simulink library "dspadpt3"  (Simulink 6.0)
settings: Solver=ode45  SolverMode=SingleTasking  StartTime=0.0  StopTime=10.0  RelTol=1e-3
undefined symbols (not defined in the file or in its folder): D, ic
libraries: dspsigattribs x27, dspmtrx3 x5, simulink x4, dspbuff3 x3, dspobslib x2, dspsigops x2, adptfiltsubsys x1, dspindex x1
settings Model: RequirementInfo=9  Creator=don  LastModifiedBy=mlongfri  ExtModeAutoUpdateStatusClock=off
settings Model: ForwardingTableString=|
  | ||__slOldName__||dspadpt3/RLS
  | Adaptive Filter||__slNewName__||dspobslib/RLS
  | Adaptive Filter||__slOldName__||dspadpt3/LMS
  | Adaptive Filter||__slNewName__||dspobslib/LMS
  | Adaptive Filter
settings DataIOCC: SignalLoggingName=logsOut
settings OptimizationCC: BooleanDataType=off
settings DebuggingCC: CheckExecutionContextPreStartOutputMsg=on  CheckExecutionContextRuntimeOutputMsg=on  SolverPrmCheckMsg=none
settings HardwareCC: TargetUnknown=on
settings ModelReferenceCC: UpdateModelReferenceTargets=IfOutOfDate
settings SFSimCC: SFSimApplyToAllLibs=on  SFSimBuildMode=Incremental

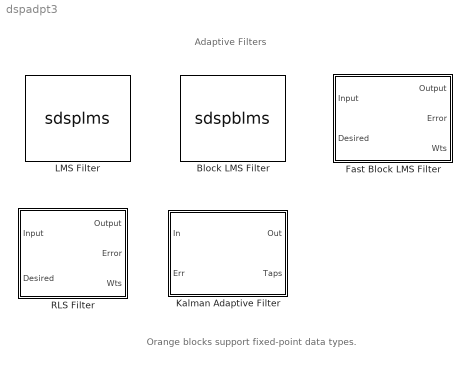
== system dspadpt3 ==
  note: Adaptive Filters
  note: Orange blocks support fixed-point data types.
  Block LMS Filter : S-Function  FunctionName=sdspblms  Parameters=L,N,stepflag,mu,leakage,addnparflag,ic,Adapt,resetflag,weights  mask(Block LMS Filter){algo=Block LMS, ShowPortLabels=off, L=32, N=32, stepflag=Dialog, mu=0.1, leakage=1.0, addnparflag=off, ic=0, Adapt=off, resetflag=None, weights=on}
      mask prompts: algo "dummy1"; ShowPortLabels "dummy2"; L "Filter length:"; N "Block size:"; stepflag "Specify step size via:"; mu "Step size (mu):"; leakage "Leakage factor (0 to 1):"; addnparflag "------------------------- Show additional parameters -------------------------"; ic "Initial value of filter weights:"; Adapt "Enable/disable adaptation via input port"; resetflag "Reset input:"; weights "Output filter weights"
      mask help:
      | Computes filter weights based on the Block LMS algorithm for filtering of the input signal. The filter weights are updated once for every block of data that is processed.
      |
      | Select the Enable/disable adaptation via input port check box to create an Adapt port on the block. When the input to this port is nonzero, the block continuously updates the filter weights. When the input to this port is zero, the filter weights remain constant.
      |
      | If the Reset port is enabled and a reset event occurs, the block resets the filter weights to their initial values.
      mask init:
      | resetflag = resetflag-1;
      | [si,so]=dspblkblklms('icon');
      | blkname = strvcat('  Block  ', '   LMS');
      mask Help: web(dspbhelp);
      mask StyleString: popup(Block LMS|Fast Block LMS),checkbox,edit,edit,popup(Dialog|Input port),edit,edit,checkbox,edit,checkbox,popup(None|Rising edge|Falling edge|Either edge|Non-zero sample),checkbox
      mask CallbackString: ||||dspblkblklms;|||dspblkblklms;||||
      mask Display:
      | disp(blkname)
      | port_label('input',si(1).port, si(1).txt);
      | port_label('input',si(2).port, si(2).txt);
      | port_label('input',si(3).port, si(3).txt);
      | port_label('input',si(4).port, si(4).txt);
      | port_label('input',si(5).port, si(5).txt);
      | 
      | port_label('output',so(1).port, so(1).txt);
      | port_label('output',so(2).port, so(2).txt);
      | port_label('output',so(3).port, so(3).txt);
  Fast Block LMS Filter : Subsystem  PropExecContextAcrossSSBoundary=on  mask(Fast Block LMS Filter){algo=Fast Block LMS, L=32, N=32, stepflag=Dialog, mu=0.1, leakage=1.0, addnparflag=off, ic=0, Adapt=off, resetflag=None, weights=on}
      mask prompts: algo "Algorithm:"; L "Filter length:"; N "Block size:"; stepflag "Specify step size via:"; mu "Step size (mu):"; leakage "Leakage factor (0 to 1):"; addnparflag "------------------------- Show additional parameters -------------------------"; ic "Inital value of filter weights:"; Adapt "Enable/disable adaptation via input port"; resetflag "Reset input:"; weights "Output filter weights"
      mask help:
      | Computes filter weights based on the Fast Block LMS algorithm for filtering of the input signal. The filter weights are updated once for every block of data that is processed. This block uses FFT for fast convolution.
      |
      | Select the Enable/disable adaptation via input port check box to create an Adapt port on the block. When the input to this port is nonzero, the block continuoulsy updates the filter weights. When the input to this port is zero, the filter weights remain constant.
      |
      | If the Reset port is enabled and a reset event occurs, the block resets the filter weights to their initial values.
      mask init:
      | if algo == 1
      | 	blkname = strvcat('  Block  ', '   LMS');
      | else
      | 	blkname = strvcat('Fast Block ', '    LMS');	
      | end
      | dspblkfblms('init');
      settings: ErrorFcn=dspblkadpterrfcn
      mask StyleString: popup(Block LMS|Fast Block LMS),edit,edit,popup(Dialog|Input port),edit,edit,checkbox,edit,checkbox,popup(None|Rising Edge|Falling Edge|Either Edge|Non-zero sample),checkbox
      mask CallbackString: |||dspblkfblms('addparams');|||dspblkfblms('addparams');||||
      mask Display: disp(blkname);
  Kalman Adaptive Filter : Subsystem  PropExecContextAcrossSSBoundary=on  mask(Kalman Adaptive Filter){Ntaps=64, Jmin=0.3, q=0.1, ic0=0, K0=0.5, Adapt=off, RstPort=None}
      mask prompts: Ntaps "FIR filter length:"; Jmin "Measurement noise variance:"; q "Process noise variance:"; ic0 "Initial value of filter taps:"; K0 "Initial error correlation matrix:"; Adapt "Adapt input"; RstPort "Reset input:"
      mask help:
      | One-step Kalman predictor algorithm for adaptive FIR filtering of input signal.
      |
      | If 'Adapt input' is checked and the Adapt signal is zero, the algorithm temporarily disables adaptation of the filter coefficients.  A non-zero signal enables filter adaptation.
      |
      | If the 'Reset input' is enabled and the Reset signal transitions appropriately, the filter coefficients are reset to the initial conditions.
      mask init:
      | if prod(size(ic0))==1, ic = ic0(ones(Ntaps,1)); else ic = ic0; end
      | if prod(size(K0))==1, K = K0.*eye(Ntaps);
      | elseif any(size(K0)==1), K = diag(K0);
      | else K=K0; end
      | dspblkadpt('init');
      mask Help: web(dspbhelp);
      mask StyleString: edit,edit,edit,edit,edit,checkbox,popup(None|Rising edge|Falling edge|Either edge|Non-zero sample)
      mask Display: disp('Kalman')
  LMS Filter : S-Function  DialogController=dspDDGCreate  DialogControllerArgs=DataTag0  FunctionName=sdsplms  Parameters=Algo,L,stepflag,mu,leakage,ic,Adapt,resetflag,weights,accum2Mode,accum2FracLength,prodOutput2Mode,prodOutput2FracLength,prodOutput3Mode,prodOutput3FracLength,prodOutput4Mode,prodOutput4FracLength,quotientMode,quotientFracLength,dtInfo.firstCoeffMode, dtInfo.firstCoeffWordLength, dtInfo.firstCoeffFracLength,dtInfo.firstCoeffMode, dtInfo.firstCoeffWordLength, dtInfo.secondCoeffFracLength,dtInfo.prodOutputMode,dtInfo.prodOutputWordLength,dtInfo.prodOutputFracLength,dtInfo.accumMode,dtInfo.accumWordLength,dtInfo.accumFracLength,dtInfo.memoryMode,dtInfo.memoryWordLength,dtInfo.memoryFracLength,dtInfo.roundingMode,dtInfo.overflowMode  mask(LMS Filter){ShowPortLabels=off, Algo=LMS, L=32, stepflag=Dialog, mu=0.1, leakage=1.0, ic=0, Adapt=off, resetflag=None, weights=on, firstCoeffMode=Same word length as first input, firstCoeffWordLength=16, firstCoeffFracLength=15, secondCoeffMode=User-defined, secondCoeffWordLength=2, secondCoeffFracLength=15, accumMode=Same as first input, accumWordLength=32, accumFracLength=20, accum2Mode=User-defined, accum2FracLength=20, prodOutputMode=Same as first input, prodOutputWordLength=32, prodOutputFracLength=20, prodOutput2Mode=User-defined, prodOutput2FracLength=20, prodOutput3Mode=User-defined, prodOutput3FracLength=20, prodOutput4Mode=User-defined, prodOutput4FracLength=20, quotientMode=User-defined, quotientFracLength=20, memoryMode=Same as first input, memoryWordLength=16, memoryFracLength=15, roundingMode=Floor, overflowMode=off, addnparflag=off}
      mask prompts: ShowPortLabels "dummy"; Algo "Algorithm:"; L "Filter length:"; stepflag "Specify step size via:"; mu "Step size (mu):"; leakage "Leakage factor (0 to 1):"; ic "Initial value of filter weights:"; Adapt "Enable/disable adaptation via input port"; resetflag "Reset input:"; weights "Output filter weights"; firstCoeffMode "Step size (mu) attributes:"; firstCoeffWordLength "Step size (mu) word length:"; firstCoeffFracLength "Step size (mu) fraction length:"; secondCoeffMode "Leakage factor attributes:"; secondCoeffWordLength "DUMMY lkg wordlength:"; secondCoeffFracLength "Leakage factor fraction length:"; accumMode "Accumulator (XTX) attributes:"; accumWordLength "Accumulator (XTX) word length:"; accumFracLength "Accumulator (XTX) fraction length:"; accum2Mode "Accumulator (WTX) attributes:"; accum2FracLength "Accumulator (WTX) fraction length:"; prodOutputMode "Product (XTX) output attributes:"; prodOutputWordLength "Product (XTX) output word length:"; prodOutputFracLength "Product (XTX) output fraction length:"; prodOutput2Mode "Product (WTX) output attributes:"; prodOutput2FracLength "Product (WTX) output fraction length:"; prodOutput3Mode "Product (mu*e) output attributes:"; prodOutput3FracLength "Product (mu*e) output fraction length:"; prodOutput4Mode "Product (Q*x) output attributes:"; prodOutput4FracLength "Product (Q*x) output fraction length:"; quotientMode "Quotient attributes:"; quotientFracLength "Quotient fraction length:"; memoryMode "State memory attributes:"; memoryWordLength "State memory word length:"; memoryFracLength "State memory fraction length:"; roundingMode "Round integer calculations toward:"; overflowMode "Saturate on integer overflow"; addnparflag "Dummy parameter"
      mask help:
      | Adapts the filter weights based on the chosen algorithm for filtering of the input signal.
      |
      | Select the Enable/disable adaptation via input port check box to create an Adapt port on the block. When the input to this port is nonzero, the block continuously updates the filter weights. When the input to this port is zero, the filter weights remain constant.
      |
      | If the Reset port is enabled and a reset event occurs, the block resets the filter weights to their initial values.
      mask init:
      | resetflag = resetflag-1;
      | ic=flipud(ic(:));
      | [si,so,disp_str,dtInfo]=dspblklms;
      | 
      | SAME_AS = 1;
      | USER_DEF = 2;
      | % prod outputs
      | if dtInfo.prodOutputMode == 0 % 'USER_DEFINED'
      | 	prodOutput2Mode = USER_DEF;
      | 	prodOutput3Mode = USER_DEF;
      | 	prodOutput4Mode = USER_DEF;
      | 	quotientMode = USER_DEF;
      | else
      | 	prodOutput2Mode = SAME_AS;
      | 	prodOutput3Mode = SAME_AS;
      | 	prodOutput4Mode = SAME_AS;
      | 	quotientMode = SAME_AS;
      | end
      | 	
      | % accums
      | if dtInfo.accumMode == 0 % 'USER_DEFINED'
      | 	accum2Mode = USER_DEF;
      | else
      | 	accum2Mode = SAME_AS;
      | end
      settings: CopyFcn=dspfixptcopycallback;
      mask Help: web(dspbhelp);
      mask StyleString: checkbox,popup(LMS|Normalized LMS|Sign-Error LMS|Sign-Data LMS|Sign-Sign LMS),edit,popup(Dialog|Input port),edit,edit,edit,checkbox,popup(None|Rising edge|Falling edge|Either edge|Non-zero sample),checkbox,popup(Same word length as first input|Specify word length|Binary point scaling|Slope and bias scaling|User-defined),edit,edit,popup(Same word length as first input|Specify word length|Binary point scaling|Slope and bias scaling|User-defined),edit,edit,popup(Same as first input|Binary point scaling|Slope and bias scaling|User-defined),edit,edit,popup(Same as first accumulator|Binary point scaling|Slope and bias scaling|User-defined),edit,popup(Same as first input|Binary point scaling|Slope and bias scaling|User-defined),edit,edit,popup(Same as first product|Binary point scaling|Slope and bias scaling|User-defined),edit,popup(Same as first product|Binary point scaling|Slope and bias scaling|User-defined),edit,popup(Same as first product|Binary point scaling|Slope and bias scaling|User-defined),edit,popup(Same as first product|Binary point scaling|Slope and bias scaling|User-defined),edit,popup(Same as first input|Binary point scaling|Slope and bias scaling|User-defined),edit,edit,popup(Floor|Nearest),checkbox,checkbox
      mask Display:
      | disp(disp_str)
      | port_label('input',si(1).port, si(1).txt);
      | port_label('input',si(2).port, si(2).txt);
      | port_label('input',si(3).port, si(3).txt);
      | port_label('input',si(4).port, si(4).txt);
      | port_label('input',si(5).port, si(5).txt);
      | 
      | port_label('output',so(1).port, so(1).txt);
      | port_label('output',so(2).port, so(2).txt);
      | port_label('output',so(3).port, so(3).txt);
  RLS Filter : Subsystem  PropExecContextAcrossSSBoundary=on  mask(RLS Adaptive filter){L=32, lambdaflag=Dialog, lambda=1.0, addnparflag=off, ic=0, delta=0.1, Adapt=off, resetflag=None, weights=on}
      mask prompts: L "Filter length:"; lambdaflag "Specify forgetting factor via:"; lambda "Forgetting factor (0 to 1):"; addnparflag "------------------------- Show additional parameters -------------------------"; ic "Initial value of filter weights:"; delta "Initial input variance estimate:"; Adapt "Enable/disable adaptation via input port"; resetflag "Reset input:"; weights "Output filter weights"
      mask help:
      | Computes filter weights based on the exponentially weighted recursive least-squares (RLS) algorithm for adaptive filtering of the input signal.
      |
      | Select the Enable/disable adaptation via input port check box to create an Adapt port on the block. When the input to this port is nonzero, the block continuoulsy updates the filter weights. When the input to this port is zero, the filter weights remain constant.
      |
      | If the Reset port is enabled and a reset event occurs, the block resets the filter weights to their initial values.
      mask init:
      | s ='RLS';
      | dspblkrls('init');
      settings: ErrorFcn=dspblkadpterrfcn
      mask StyleString: edit,popup(Dialog|Input port),edit,checkbox,edit,edit,checkbox,popup(None|Rising edge|Falling edge|Either edge|Non-zero sample),checkbox
      mask CallbackString: |dspblkrls('addparams');||dspblkrls('addparams');|||||
      mask Display: disp(s);

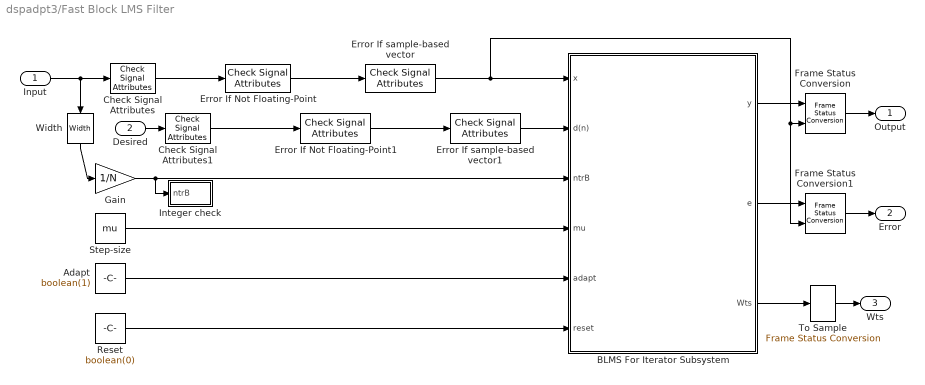
== system dspadpt3/Fast Block LMS Filter ==
  Input : Inport  LatchInput=off
  Desired : Inport  Port=2  LatchInput=off
  Adapt : Constant  Value=boolean(1)
  BLMS For Iterator Subsystem : Subsystem  TreatAsAtomicUnit=on  PropExecContextAcrossSSBoundary=on  mask{algo_for=Fast Block LMS, stepflag_for=off, weights_for=on}
      mask prompts: algo_for "Algorithm:"; stepflag_for "Input step size via port:"; weights_for "Send filter weights to output:"
      mask init:
      | dspblkfblmsfor;
      mask StyleString: popup(Block LMS|Fast Block LMS),checkbox,checkbox
  Check Signal Attributes : dspsigattribs/Check Signal Attributes  SigAttribCheckMethod=Matches attributes exactly  Complexity=Ignore  Frame=Ignore  DimsCheckMethod=Is...  Dimensions=Full matrix (2-D)  DatatypeCheckMethod=Ignore  DatatypeGeneral=Boolean  DtypeFloatSpecific=Any floating-point  DtypeFixedSpecific=Any fixed-point  DtypeIntSpecific=Any integer  SampleMode=Ignore
  Check Signal Attributes1 : dspsigattribs/Check Signal Attributes  SigAttribCheckMethod=Matches attributes exactly  Complexity=Ignore  Frame=Ignore  DimsCheckMethod=Is...  Dimensions=Full matrix (2-D)  DatatypeCheckMethod=Ignore  DatatypeGeneral=Boolean  DtypeFloatSpecific=Any floating-point  DtypeFixedSpecific=Any fixed-point  DtypeIntSpecific=Any integer  SampleMode=Ignore
  Error If Not Floating-Point : dspsigattribs/Check Signal Attributes  SigAttribCheckMethod=Does not match attributes exactly  Complexity=Ignore  Frame=Ignore  DimsCheckMethod=Ignore  Dimensions=1-D  DatatypeCheckMethod=Is...  DatatypeGeneral=Floating-point  DtypeFloatSpecific=Any floating-point  DtypeFixedSpecific=Any fixed-point  DtypeIntSpecific=Any integer  SampleMode=Ignore
  Error If Not Floating-Point1 : dspsigattribs/Check Signal Attributes  SigAttribCheckMethod=Does not match attributes exactly  Complexity=Ignore  Frame=Ignore  DimsCheckMethod=Ignore  Dimensions=1-D  DatatypeCheckMethod=Is...  DatatypeGeneral=Floating-point  DtypeFloatSpecific=Any floating-point  DtypeFixedSpecific=Any fixed-point  DtypeIntSpecific=Any integer  SampleMode=Ignore
  Error If sample-based vector : dspsigattribs/Check Signal Attributes  SigAttribCheckMethod=Matches attributes exactly  Complexity=Ignore  Frame=Sample-based  DimsCheckMethod=Is...  Dimensions=Vector (1-D or 2-D)  DatatypeCheckMethod=Ignore  DatatypeGeneral=Boolean  DtypeFloatSpecific=Any floating-point  DtypeFixedSpecific=Any fixed-point  DtypeIntSpecific=Any integer  SampleMode=Ignore
  Error If sample-based vector1 : dspsigattribs/Check Signal Attributes  SigAttribCheckMethod=Matches attributes exactly  Complexity=Ignore  Frame=Sample-based  DimsCheckMethod=Is...  Dimensions=Vector (1-D or 2-D)  DatatypeCheckMethod=Ignore  DatatypeGeneral=Boolean  DtypeFloatSpecific=Any floating-point  DtypeFixedSpecific=Any fixed-point  DtypeIntSpecific=Any integer  SampleMode=Ignore
  Frame Status Conversion : dspsigattribs/Frame Status Conversion  growRefPort=on  outframe=Sample-based
  Frame Status Conversion1 : dspsigattribs/Frame Status Conversion  growRefPort=on  outframe=Sample-based
  Gain : Gain  Gain=1/N  SaturateOnIntegerOverflow=on
  Integer check : Subsystem  PropExecContextAcrossSSBoundary=on
  Reset : Constant  Value=boolean(0)
  Step-size : Constant  Value=mu
  To Sample : dspsigattribs/Frame Status Conversion  growRefPort=off  outframe=Sample-based
  Width : Width  Orientation=down
  Output : Outport
  Error : Outport  Port=2
  Wts : Outport  Port=3
  wires:
  Step-size/1 -> BLMS For Iterator Subsystem/4(mu)
  Check Signal Attributes1/1 -> Error If Not Floating-Point1/1
  Check Signal Attributes/1 -> Error If Not Floating-Point/1
  To Sample/1 -> Wts/1
  BLMS For Iterator Subsystem/3(Wts) -> To Sample/1
  Desired/1 -> Check Signal Attributes1/1
  Input/1 -> Check Signal Attributes/1, Width/1
  Gain/1 -> Integer check/1(ntrB), BLMS For Iterator Subsystem/3(ntrB)
  Width/1 -> Gain/1
  Reset/1 -> BLMS For Iterator Subsystem/6(reset)
  Adapt/1 -> BLMS For Iterator Subsystem/5(adapt)
  BLMS For Iterator Subsystem/1(y) -> Frame Status Conversion/1
  Frame Status Conversion/1 -> Output/1
  BLMS For Iterator Subsystem/2(e) -> Frame Status Conversion1/1
  Frame Status Conversion1/1 -> Error/1
  Error If Not Floating-Point/1 -> Error If sample-based vector/1
  Error If Not Floating-Point1/1 -> Error If sample-based vector1/1
  Error If sample-based vector/1 -> BLMS For Iterator Subsystem/1(x), Frame Status Conversion/2, Frame Status Conversion1/2
  Error If sample-based vector1/1 -> BLMS For Iterator Subsystem/2(d(n))

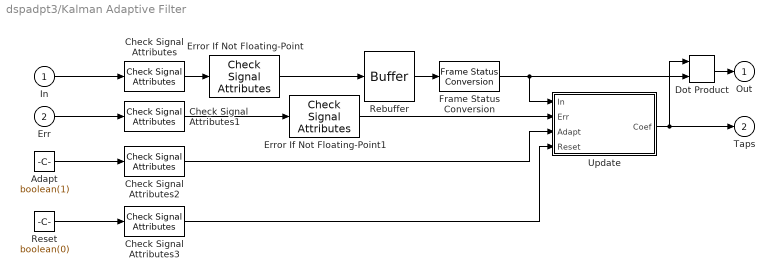
== system dspadpt3/Kalman Adaptive Filter ==
  In : Inport  LatchInput=off
  Err : Inport  Port=2  LatchInput=off
  Adapt : Constant  Value=boolean(1)
  Check Signal Attributes{,1..3} (4 alike) : dspsigattribs/Check Signal Attributes  SigAttribCheckMethod=Does not match attributes exactly  Complexity=Ignore  Frame=Sample-based  DimsCheckMethod=Is...  Dimensions=Scalar (1-D or 2-D)  DatatypeCheckMethod=Ignore  DatatypeGeneral=Boolean  DtypeFloatSpecific=Any floating-point  DtypeFixedSpecific=Any fixed-point  DtypeIntSpecific=Any integer  SampleMode=Ignore
  Dot Product : simulink/Math Operations/Dot Product  OutDataType=sfix(16)  OutScaling=2^-10  DoSatur=off
  Error If Not Floating-Point : dspsigattribs/Check Signal Attributes  SigAttribCheckMethod=Does not match attributes exactly  Complexity=Ignore  Frame=Ignore  DimsCheckMethod=Ignore  Dimensions=1-D  DatatypeCheckMethod=Is...  DatatypeGeneral=Floating-point  DtypeFloatSpecific=Any floating-point  DtypeFixedSpecific=Any fixed-point  DtypeIntSpecific=Any integer  SampleMode=Ignore
  Error If Not Floating-Point1 : dspsigattribs/Check Signal Attributes  SigAttribCheckMethod=Does not match attributes exactly  Complexity=Ignore  Frame=Ignore  DimsCheckMethod=Ignore  Dimensions=1-D  DatatypeCheckMethod=Is...  DatatypeGeneral=Floating-point  DtypeFloatSpecific=Any floating-point  DtypeFixedSpecific=Any fixed-point  DtypeIntSpecific=Any integer  SampleMode=Ignore
  Frame Status Conversion : dspsigattribs/Frame Status Conversion  growRefPort=off  outframe=Sample-based
  Rebuffer : dspbuff3/Buffer  N=Ntaps  V=Ntaps-1  ic=0
  Reset : Constant  Value=boolean(0)
  Update : Subsystem  PropExecContextAcrossSSBoundary=on
  Out : Outport  InitialOutput=0
  Taps : Outport  Port=2  InitialOutput=0
  wires:
  Err/1 -> Check Signal Attributes1/1
  In/1 -> Check Signal Attributes/1
  Adapt/1 -> Check Signal Attributes2/1
  Dot Product/1 -> Out/1
  Rebuffer/1 -> Frame Status Conversion/1
  Update/1(Coef) -> Taps/1, Dot Product/1
  Check Signal Attributes1/1 -> Error If Not Floating-Point1/1
  Check Signal Attributes/1 -> Error If Not Floating-Point/1
  Check Signal Attributes2/1 -> Update/3(Adapt)
  Frame Status Conversion/1 -> Update/1(In), Dot Product/2
  Reset/1 -> Check Signal Attributes3/1
  Check Signal Attributes3/1 -> Update/4(Reset)
  Error If Not Floating-Point/1 -> Rebuffer/1
  Error If Not Floating-Point1/1 -> Update/2(Err)

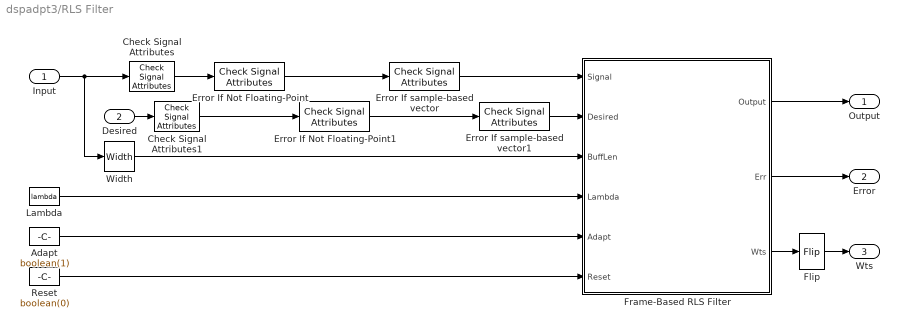
== system dspadpt3/RLS Filter ==
  Input : Inport  LatchInput=off
  Desired : Inport  Port=2  LatchInput=off
  Adapt : Constant  Value=boolean(1)
  Check Signal Attributes : dspsigattribs/Check Signal Attributes  SigAttribCheckMethod=Matches attributes exactly  Complexity=Ignore  Frame=Ignore  DimsCheckMethod=Is...  Dimensions=Full matrix (2-D)  DatatypeCheckMethod=Ignore  DatatypeGeneral=Boolean  DtypeFloatSpecific=Any floating-point  DtypeFixedSpecific=Any fixed-point  DtypeIntSpecific=Any integer  SampleMode=Ignore
  Check Signal Attributes1 : dspsigattribs/Check Signal Attributes  SigAttribCheckMethod=Matches attributes exactly  Complexity=Ignore  Frame=Ignore  DimsCheckMethod=Is...  Dimensions=Full matrix (2-D)  DatatypeCheckMethod=Ignore  DatatypeGeneral=Boolean  DtypeFloatSpecific=Any floating-point  DtypeFixedSpecific=Any fixed-point  DtypeIntSpecific=Any integer  SampleMode=Ignore
  Error If Not Floating-Point : dspsigattribs/Check Signal Attributes  SigAttribCheckMethod=Does not match attributes exactly  Complexity=Ignore  Frame=Ignore  DimsCheckMethod=Ignore  Dimensions=1-D  DatatypeCheckMethod=Is...  DatatypeGeneral=Floating-point  DtypeFloatSpecific=Any floating-point  DtypeFixedSpecific=Any fixed-point  DtypeIntSpecific=Any integer  SampleMode=Ignore
  Error If Not Floating-Point1 : dspsigattribs/Check Signal Attributes  SigAttribCheckMethod=Does not match attributes exactly  Complexity=Ignore  Frame=Ignore  DimsCheckMethod=Ignore  Dimensions=1-D  DatatypeCheckMethod=Is...  DatatypeGeneral=Floating-point  DtypeFloatSpecific=Any floating-point  DtypeFixedSpecific=Any fixed-point  DtypeIntSpecific=Any integer  SampleMode=Ignore
  Error If sample-based vector : dspsigattribs/Check Signal Attributes  SigAttribCheckMethod=Matches attributes exactly  Complexity=Ignore  Frame=Sample-based  DimsCheckMethod=Is...  Dimensions=Vector (1-D or 2-D)  DatatypeCheckMethod=Ignore  DatatypeGeneral=Boolean  DtypeFloatSpecific=Any floating-point  DtypeFixedSpecific=Any fixed-point  DtypeIntSpecific=Any integer  SampleMode=Ignore
  Error If sample-based vector1 : dspsigattribs/Check Signal Attributes  SigAttribCheckMethod=Matches attributes exactly  Complexity=Ignore  Frame=Sample-based  DimsCheckMethod=Is...  Dimensions=Vector (1-D or 2-D)  DatatypeCheckMethod=Ignore  DatatypeGeneral=Boolean  DtypeFloatSpecific=Any floating-point  DtypeFixedSpecific=Any fixed-point  DtypeIntSpecific=Any integer  SampleMode=Ignore
  Flip : dspindex/Flip  dim=Columns
  Frame-Based RLS Filter : Subsystem  TreatAsAtomicUnit=on  PropExecContextAcrossSSBoundary=on  mask{weights_for=on}
      mask prompts: weights_for "Send filter weights to output:"
      mask init:
      | dspblkrlsfor;
  Lambda : Constant  Value=lambda
  Reset : Constant  Value=boolean(0)
  Width : Width
  Output : Outport
  Error : Outport  Port=2
  Wts : Outport  Port=3
  wires:
  Flip/1 -> Wts/1
  Frame-Based RLS Filter/3(Wts) -> Flip/1
  Frame-Based RLS Filter/2(Err) -> Error/1
  Reset/1 -> Frame-Based RLS Filter/6(Reset)
  Frame-Based RLS Filter/1(Output) -> Output/1
  Desired/1 -> Check Signal Attributes1/1
  Input/1 -> Width/1, Check Signal Attributes/1
  Width/1 -> Frame-Based RLS Filter/3(BuffLen)
  Adapt/1 -> Frame-Based RLS Filter/5(Adapt)
  Lambda/1 -> Frame-Based RLS Filter/4(Lambda)
  Check Signal Attributes/1 -> Error If Not Floating-Point/1
  Check Signal Attributes1/1 -> Error If Not Floating-Point1/1
  Error If Not Floating-Point/1 -> Error If sample-based vector/1
  Error If Not Floating-Point1/1 -> Error If sample-based vector1/1
  Error If sample-based vector/1 -> Frame-Based RLS Filter/1(Signal)
  Error If sample-based vector1/1 -> Frame-Based RLS Filter/2(Desired)

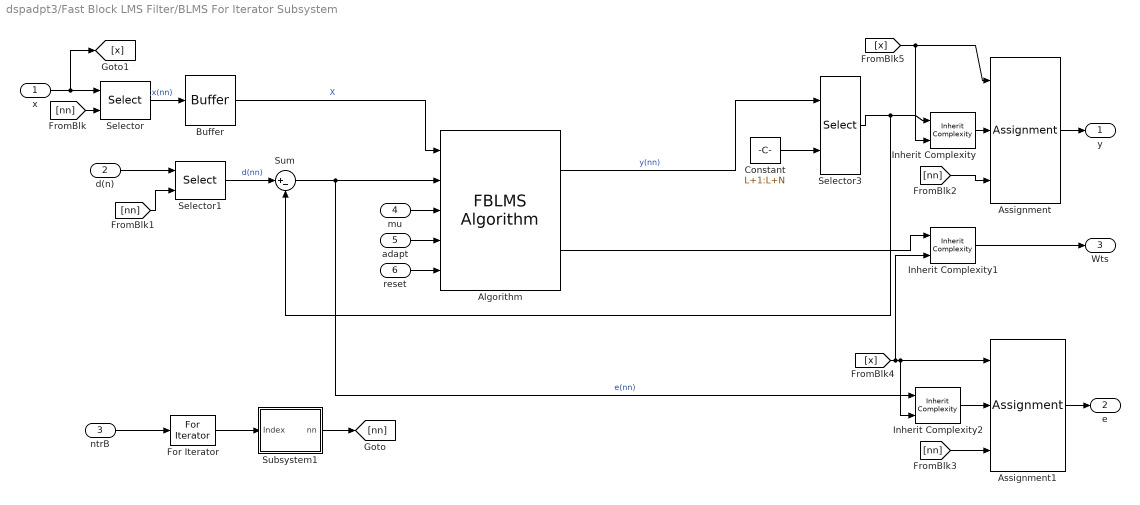
== system dspadpt3/Fast Block LMS Filter/BLMS For Iterator Subsystem ==
  x : Inport  LatchInput=off
  d(n) : Inport  Port=2  LatchInput=off
  ntrB : Inport  Port=3  LatchInput=off
  mu : Inport  Port=4  LatchInput=off
  adapt : Inport  Port=5  LatchInput=off
  reset : Inport  Port=6  LatchInput=off
  Algorithm : adptfiltsubsys/FBLMS Algorithm  weights_algo=on
  Assignment : Assignment  ElementSrc=External
  Assignment1 : Assignment  ElementSrc=External
  Buffer : dspbuff3/Buffer  N=L+N  V=L  ic=0
  Constant : Constant  Value=L+1:L+N
  For Iterator : ForIterator  IterationSource=external  IterationVariableDataType=double
  Inherit Complexity : dspsigattribs/Inherit Complexity
  Inherit Complexity1 : dspsigattribs/Inherit Complexity
  Inherit Complexity2 : dspsigattribs/Inherit Complexity
  Selector : Selector  ElementSrc=External  Elements=[1 3]
  Selector1 : Selector  ElementSrc=External  Elements=[1 3]
  Selector3 : Selector  ElementSrc=External  Elements=[1 3]
  Subsystem1 : Subsystem  PropExecContextAcrossSSBoundary=on
  Sum : Sum  Inputs=|+-  SaturateOnIntegerOverflow=on
  y : Outport
  e : Outport  Port=2
  Wts : Outport  Port=3
  wires:
  Algorithm/2 -> Inherit Complexity1/1
  adapt/1 -> Algorithm/4
  mu/1 -> Algorithm/3
  Buffer/1 -> Algorithm/1  "X"
  Inherit Complexity1/1 -> Wts/1
  Inherit Complexity2/1 -> Assignment1/2
  Inherit Complexity/1 -> Assignment/2
  Sum/1 -> Algorithm/2, Inherit Complexity2/1  "e(nn)"
  Selector1/1 -> Sum/1  "d(nn)"
  [nn] -> Assignment1/3
  Assignment1/1 -> e/1
  ntrB/1 -> For Iterator/1
  For Iterator/1 -> Subsystem1/1(Index)
  Assignment/1 -> y/1
  x/1 -> Selector/1, [x]
  [nn] -> Selector/2
  d(n)/1 -> Selector1/1
  [nn] -> Selector1/2
  Subsystem1/1(nn) -> [nn]
  Selector/1 -> Buffer/1  "x(nn)"
  reset/1 -> Algorithm/5
  Constant/1 -> Selector3/2
  Selector3/1 -> Sum/2, Inherit Complexity/1
  Algorithm/1 -> Selector3/1  "y(nn)"
  [nn] -> Assignment/3
  [x] -> Inherit Complexity1/2, Assignment1/1, Inherit Complexity2/2
  [x] -> Assignment/1, Inherit Complexity/2

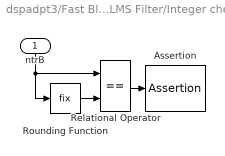
== system dspadpt3/Fast Block LMS Filter/Integer check ==
  ntrB : Inport  Orientation=down  LatchInput=off
  Assertion : Assertion  AssertionFailFcn=error('The input frame length is not an integer multiple of the Block length');
  Relational Operator : RelationalOperator  Operator===  LogicOutDataTypeMode=Boolean
  Rounding Function : Rounding  Operator=fix
  wires:
  Rounding Function/1 -> Relational Operator/2
  Relational Operator/1 -> Assertion/1
  ntrB/1 -> Relational Operator/1, Rounding Function/1

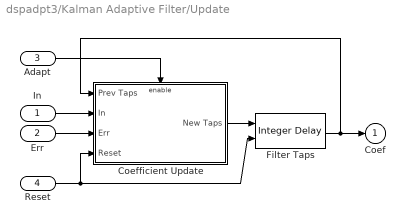
== system dspadpt3/Kalman Adaptive Filter/Update ==
  In : Inport  LatchInput=off
  Err : Inport  Port=2  LatchInput=off
  Adapt : Inport  Port=3  LatchInput=off
  Reset : Inport  Port=4  LatchInput=off
  Coefficient Update : Subsystem  TreatAsAtomicUnit=on  PropExecContextAcrossSSBoundary=on
  Filter Taps : dspobslib/Integer Delay  delay=1  ic=ic  reset_popup=Non-zero sample
  Coef : Outport  InitialOutput=0
  wires:
  Filter Taps/1 -> Coef/1, Coefficient Update/1(Prev Taps)
  Coefficient Update/1(New Taps) -> Filter Taps/1
  In/1 -> Coefficient Update/2(In)
  Err/1 -> Coefficient Update/3(Err)
  Adapt/1 -> Coefficient Update/Enable
  Reset/1 -> Filter Taps/2, Coefficient Update/4(Reset)

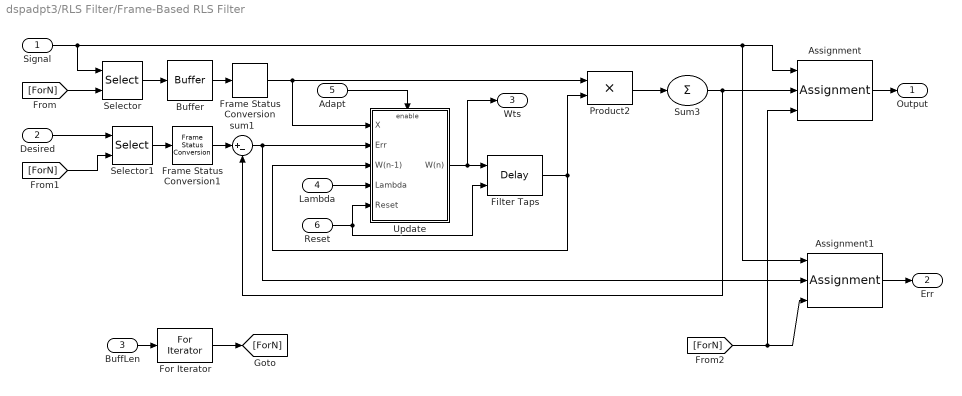
== system dspadpt3/RLS Filter/Frame-Based RLS Filter ==
  Signal : Inport  LatchInput=off
  Desired : Inport  Port=2  LatchInput=off
  BuffLen : Inport  Port=3  LatchInput=off
  Lambda : Inport  Port=4  LatchInput=off
  Adapt : Inport  Port=5  LatchInput=off
  Reset : Inport  Port=6  LatchInput=off
  Assignment : Assignment  ElementSrc=External  Rows=-1  ColumnSrc=External
  Assignment1 : Assignment  ElementSrc=External  Rows=-1  ColumnSrc=External
  Buffer : dspbuff3/Buffer  N=L  V=L-1  ic=0
  Filter Taps : dspsigops/Delay  dly_unit=Samples  delay=1  ic_detail=on  dif_ic_for_ch=off  dif_ic_for_dly=off  ic=flipud(ic(:))  reset_popup=Non-zero sample
  For Iterator : ForIterator  IterationSource=external  IterationLimit=4
  Frame Status Conversion : dspsigattribs/Frame Status Conversion  growRefPort=off  outframe=Sample-based
  Frame Status Conversion1 : dspsigattribs/Frame Status Conversion  growRefPort=off  outframe=Sample-based
  Product2 : Product  SaturateOnIntegerOverflow=on
  Selector : Selector  ElementSrc=External  Elements=[1 3]
  Selector1 : Selector  ElementSrc=External  Elements=[1 3]
  Sum3 : Sum  Inputs=1  SaturateOnIntegerOverflow=on
  Update : Subsystem  PropExecContextAcrossSSBoundary=on
  sum1 : Sum  Inputs=|+-  SaturateOnIntegerOverflow=on  InputSameDT=on
  Output : Outport
  Err : Outport  Port=2
  Wts : Outport  Port=3
  wires:
  Assignment1/1 -> Err/1
  Selector1/1 -> Frame Status Conversion1/1
  [ForN] -> Selector1/2
  [ForN] -> Selector/2
  For Iterator/1 -> [ForN]
  Selector/1 -> Buffer/1
  BuffLen/1 -> For Iterator/1
  Desired/1 -> Selector1/1
  Assignment/1 -> Output/1
  Signal/1 -> Selector/1, Assignment/1, Assignment1/1
  Buffer/1 -> Frame Status Conversion/1
  Update/1(W(n)) -> Filter Taps/1, Wts/1
  Filter Taps/1 -> Product2/2, Update/3(W(n-1))
  Product2/1 -> Sum3/1
  Sum3/1 -> sum1/2, Assignment/2
  sum1/1 -> Update/2(Err), Assignment1/2
  Reset/1 -> Filter Taps/2, Update/5(Reset)
  [ForN] -> Assignment/3, Assignment1/3
  Adapt/1 -> Update/Enable
  Frame Status Conversion/1 -> Product2/1, Update/1(X)
  Frame Status Conversion1/1 -> sum1/1
  Lambda/1 -> Update/4(Lambda)

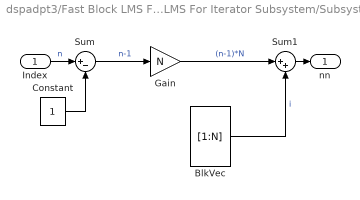
== system dspadpt3/Fast Block LMS Filter/BLMS For Iterator Subsystem/Subsystem1 ==
  Index : Inport  LatchInput=off
  BlkVec : Constant  Value=[1:N]
  Constant : Constant
  Gain : Gain  Gain=N  SaturateOnIntegerOverflow=on
  Sum : Sum  Inputs=|+-  SaturateOnIntegerOverflow=on
  Sum1 : Sum  Inputs=|++  SaturateOnIntegerOverflow=on
  nn : Outport
  wires:
  Sum1/1 -> nn/1
  Index/1 -> Sum/1  "n"
  BlkVec/1 -> Sum1/2  "i"
  Gain/1 -> Sum1/1  "(n-1)*N"
  Sum/1 -> Gain/1  "n-1"
  Constant/1 -> Sum/2

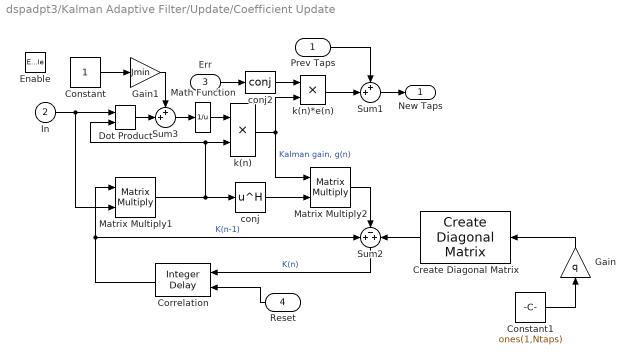
== system dspadpt3/Kalman Adaptive Filter/Update/Coefficient Update ==
  Prev Taps : Inport  LatchInput=off
  In : Inport  Port=2  LatchInput=off
  Err : Inport  Port=3  LatchInput=off
  Reset : Inport  Orientation=left  Port=4  LatchInput=off
  Enable : EnablePort  ZeroCross=off
  Constant : Constant
  Constant1 : Constant  Value=ones(1,Ntaps)
  Correlation : dspobslib/Integer Delay  Orientation=left  delay=1  ic=K  reset_popup=Either edge
  Create Diagonal Matrix : dspmtrx3/Create Diagonal Matrix  Orientation=left
  Dot Product : simulink/Math Operations/Dot Product
  Gain : Gain  Orientation=up  Gain=q  SaturateOnIntegerOverflow=on
  Gain1 : Gain  Gain=Jmin  SaturateOnIntegerOverflow=on
  Math Function : Math  Operator=reciprocal  SaturateOnIntegerOverflow=on
  Matrix Multiply1 : dspmtrx3/Matrix Multiply  numInputPorts=2  OptimizationLevel=None
  Matrix Multiply2 : dspmtrx3/Matrix Multiply  numInputPorts=2  OptimizationLevel=None
  Sum1 : Sum  Inputs=++|  SaturateOnIntegerOverflow=on  InputSameDT=on
  Sum2 : Sum  Orientation=down  Inputs=+-+  SaturateOnIntegerOverflow=on  InputSameDT=on
  Sum3 : Sum  Inputs=++|  SaturateOnIntegerOverflow=on  InputSameDT=on
  conj : Math  Operator=hermitian  SaturateOnIntegerOverflow=on
  conj2 : Math  Operator=conj  SaturateOnIntegerOverflow=on
  k(n) : Product  SaturateOnIntegerOverflow=on  InputSameDT=on
  k(n)*e(n) : Product  SaturateOnIntegerOverflow=on  InputSameDT=on
  New Taps : Outport  InitialOutput=ic
  wires:
  Gain1/1 -> Sum3/1
  Gain/1 -> Create Diagonal Matrix/1
  In/1 -> Matrix Multiply1/2, Dot Product/1
  Create Diagonal Matrix/1 -> Sum2/3
  Sum2/1 -> Correlation/1  "K(n)"
  Correlation/1 -> Sum2/1, Matrix Multiply1/1  "K(n-1)"
  Constant/1 -> Gain1/1
  Dot Product/1 -> Sum3/2
  Matrix Multiply2/1 -> Sum2/2
  conj/1 -> Matrix Multiply2/2
  Matrix Multiply1/1 -> conj/1, k(n)/2, Dot Product/2
  Sum3/1 -> Math Function/1
  k(n)/1 -> Matrix Multiply2/1, k(n)*e(n)/2  "Kalman gain, g(n)"
  Err/1 -> conj2/1
  conj2/1 -> k(n)*e(n)/1
  k(n)*e(n)/1 -> Sum1/2
  Prev Taps/1 -> Sum1/1
  Sum1/1 -> New Taps/1
  Math Function/1 -> k(n)/1
  Constant1/1 -> Gain/1
  Reset/1 -> Correlation/2

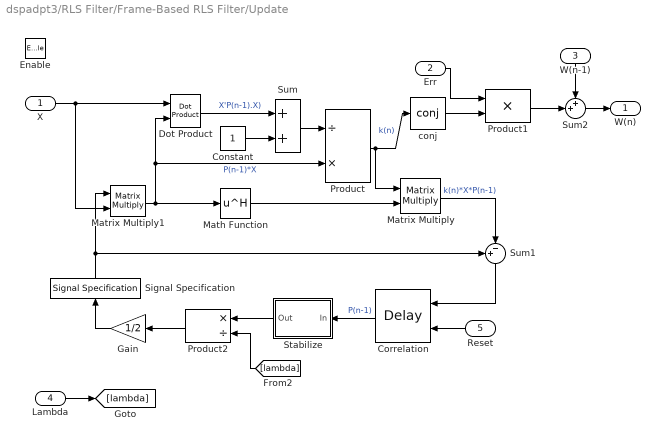
== system dspadpt3/RLS Filter/Frame-Based RLS Filter/Update ==
  X : Inport  LatchInput=off
  Err : Inport  Port=2  LatchInput=off
  W(n-1) : Inport  Orientation=down  Port=3  LatchInput=off
  Lambda : Inport  Port=4  LatchInput=off
  Reset : Inport  Orientation=left  Port=5  LatchInput=off
  Enable : EnablePort
  Constant : Constant
  Correlation : dspsigops/Delay  Orientation=left  dly_unit=Samples  delay=1  ic_detail=on  dif_ic_for_ch=on  dif_ic_for_dly=off  ic=eye(L)./delta  reset_popup=Non-zero sample
  Dot Product : simulink/Math Operations/Dot Product
  Gain : Gain  Orientation=left  Gain=1/2  SaturateOnIntegerOverflow=on
  Math Function : Math  Operator=hermitian  SaturateOnIntegerOverflow=on
  Matrix Multiply : dspmtrx3/Matrix Multiply  numInputPorts=2  OptimizationLevel=None
  Matrix Multiply1 : dspmtrx3/Matrix Multiply  numInputPorts=2  OptimizationLevel=None
  Product : Product  Inputs=/*  SaturateOnIntegerOverflow=on
  Product1 : Product  SaturateOnIntegerOverflow=on
  Product2 : Product  Orientation=left  Inputs=*/  SaturateOnIntegerOverflow=on
  Signal Specification : simulink/Signal Attributes/Signal Specification  Orientation=up  D=[L,L]  Ts=-1  DataType=auto  OutDataType=sfix(16)  OutScaling=2^0
      settings: SignalType=auto  SamplingMode=auto
  Stabilize : Subsystem  Orientation=left  PropExecContextAcrossSSBoundary=on
  Sum : Sum  SaturateOnIntegerOverflow=on
  Sum1 : Sum  Orientation=down  Inputs=+-|  SaturateOnIntegerOverflow=on
  Sum2 : Sum  Inputs=++|  SaturateOnIntegerOverflow=on
  conj : Math  Operator=conj  SaturateOnIntegerOverflow=on
  W(n) : Outport
  wires:
  Dot Product/1 -> Sum/1  "X'P(n-1).X)"
  Sum/1 -> Product/1
  Matrix Multiply1/1 -> Dot Product/2, Product/2, Math Function/1  "P(n-1)*X"
  Product/1 -> Matrix Multiply/1, conj/1  "k(n)"
  Math Function/1 -> Matrix Multiply/2
  Matrix Multiply/1 -> Sum1/2  "k(n)*X*P(n-1)"
  Sum1/1 -> Correlation/1
  Product1/1 -> Sum2/2
  W(n-1)/1 -> Sum2/1
  Err/1 -> Product1/1
  X/1 -> Dot Product/1, Matrix Multiply1/2
  Sum2/1 -> W(n)/1
  Signal Specification/1 -> Matrix Multiply1/1, Sum1/1
  Reset/1 -> Correlation/2
  Correlation/1 -> Stabilize/1(In)  "P(n-1)"
  Gain/1 -> Signal Specification/1
  Lambda/1 -> [lambda]
  Product2/1 -> Gain/1
  Stabilize/1(Out) -> Product2/1
  [lambda] -> Product2/2
  conj/1 -> Product1/2
  Constant/1 -> Sum/2

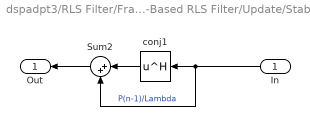
== system dspadpt3/RLS Filter/Frame-Based RLS Filter/Update/Stabilize ==
  In : Inport  Orientation=left  LatchInput=off
  Sum2 : Sum  Orientation=left  Inputs=|++  SaturateOnIntegerOverflow=on  InputSameDT=on
  conj1 : Math  Orientation=left  Operator=hermitian  SaturateOnIntegerOverflow=on
  Out : Outport  Orientation=left
  wires:
  In/1 -> conj1/1, Sum2/2  "P(n-1)/Lambda"
  conj1/1 -> Sum2/1
  Sum2/1 -> Out/1
